simulink model "fmpc_simulation_3modelle"  (R2022b)
settings: Solver=VariableStepAuto  StartTime=0.0  StopTime=T  RelTol=1e-7
undefined symbols (not defined in the file): Am, b, Bm, c_1, c_2, C_hilf, Cm, D, dt, F1, F2, F3, fuzzy_menge, H1, H2, H3, PhiU1, PhiU2, PhiU3, PhiZ1, PhiZ2, PhiZ3, Qy1, Qy2, Qy3
settings Model: Creator=benja  LastModifiedBy=benja

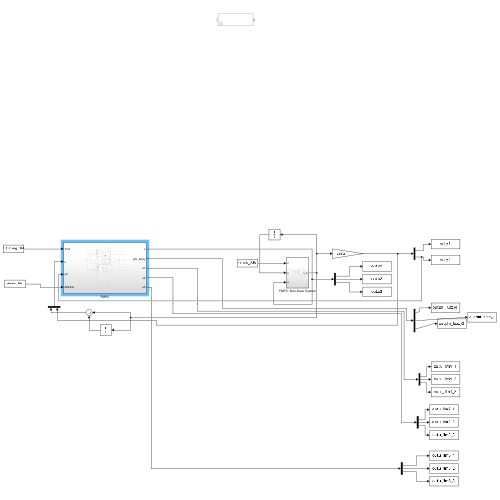
[thumbnail: Simulink's stored preview of the top-level diagram]
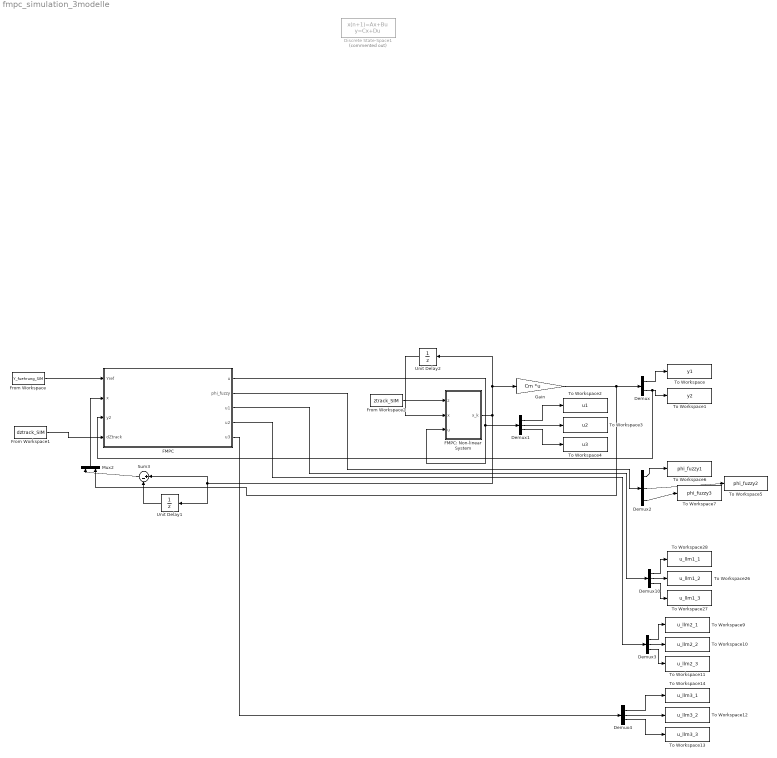
== system fmpc_simulation_3modelle ==
  Demux : Demux  Outputs=2
  Demux{1..4,10} (5 alike) : Demux  Outputs=3
  Discrete State-Space1 : DiscreteStateSpace  Commented=on  A=Am  B=Bm  C=C_hilf  D=D  SampleTime=dt
  FMPC : Subsystem
  FMPC: Non-linear System : Subsystem
  From Workspace : FromWorkspace  VariableName=Y_fuehrung_SIM  OutDataTypeStr=double  SampleTime=dt
  From Workspace1 : FromWorkspace  VariableName=dztrack_SIM  OutDataTypeStr=double  SampleTime=dt
  From Workspace2 : FromWorkspace  VariableName=ztrack_SIM  OutDataTypeStr=double  SampleTime=dt
  Gain : Gain  Gain=Cm  Multiplication=Matrix(K*u)
  Mux2 : Mux  Inputs=2
  Sum3 : Sum  Inputs=|+-
  To Workspace : ToWorkspace  VariableName=y1  SampleTime=-1
      settings: Save2DSignal=2-D array (concatenate along first dimension)
  To Workspace1 : ToWorkspace  VariableName=y2  SampleTime=-1
      settings: Save2DSignal=2-D array (concatenate along first dimension)
  To Workspace10 : ToWorkspace  VariableName=u_llm2_2  SampleTime=-1
      settings: Save2DSignal=2-D array (concatenate along first dimension)
  To Workspace11 : ToWorkspace  VariableName=u_llm2_3  SampleTime=-1
      settings: Save2DSignal=2-D array (concatenate along first dimension)
  To Workspace12 : ToWorkspace  VariableName=u_llm3_2  SampleTime=-1
      settings: Save2DSignal=2-D array (concatenate along first dimension)
  To Workspace13 : ToWorkspace  VariableName=u_llm3_3  SampleTime=-1
      settings: Save2DSignal=2-D array (concatenate along first dimension)
  To Workspace14 : ToWorkspace  VariableName=u_llm3_1  SampleTime=-1
      settings: Save2DSignal=2-D array (concatenate along first dimension)
  To Workspace2 : ToWorkspace  VariableName=u1  SampleTime=-1
      settings: Save2DSignal=2-D array (concatenate along first dimension)
  To Workspace26 : ToWorkspace  VariableName=u_llm1_2  SampleTime=-1
      settings: Save2DSignal=2-D array (concatenate along first dimension)
  To Workspace27 : ToWorkspace  VariableName=u_llm1_3  SampleTime=-1
      settings: Save2DSignal=2-D array (concatenate along first dimension)
  To Workspace28 : ToWorkspace  VariableName=u_llm1_1  SampleTime=-1
      settings: Save2DSignal=2-D array (concatenate along first dimension)
  To Workspace3 : ToWorkspace  VariableName=u2  SampleTime=-1
      settings: Save2DSignal=2-D array (concatenate along first dimension)
  To Workspace4 : ToWorkspace  VariableName=u3  SampleTime=-1
      settings: Save2DSignal=2-D array (concatenate along first dimension)
  To Workspace5 : ToWorkspace  VariableName=phi_fuzzy2  SampleTime=-1
      settings: Save2DSignal=2-D array (concatenate along first dimension)
  To Workspace6 : ToWorkspace  VariableName=phi_fuzzy1  SampleTime=-1
      settings: Save2DSignal=2-D array (concatenate along first dimension)
  To Workspace7 : ToWorkspace  VariableName=phi_fuzzy3  SampleTime=-1
      settings: Save2DSignal=2-D array (concatenate along first dimension)
  To Workspace9 : ToWorkspace  VariableName=u_llm2_1  SampleTime=-1
      settings: Save2DSignal=2-D array (concatenate along first dimension)
  Unit Delay1 : UnitDelay  SampleTime=-1  HasFrameUpgradeWarning=on
  Unit Delay2 : UnitDelay  SampleTime=-1  HasFrameUpgradeWarning=on
  wires:
  Demux/1 -> To Workspace/1
  Demux1/1 -> To Workspace2/1
  Demux1/2 -> To Workspace3/1
  Unit Delay1/1 -> Sum3/2
  Gain/1 -> Demux/1, Mux2/2
  Sum3/1 -> Mux2/1
  Demux1/3 -> To Workspace4/1
  FMPC: Non-linear System/1(x_k) -> Unit Delay2/1, Gain/1, Sum3/1, Unit Delay1/1
  Unit Delay2/1 -> FMPC: Non-linear System/2(x)
  FMPC/1(u) -> FMPC: Non-linear System/3(u), Demux1/1
  From Workspace/1 -> FMPC/1(Yref)
  Mux2/1 -> FMPC/2(x)
  FMPC/2(phi_fuzzy) -> Demux2/1
  Demux2/1 -> To Workspace6/1
  Demux2/2 -> To Workspace5/1
  Demux2/3 -> To Workspace7/1
  Demux/2 -> FMPC/3(y2), To Workspace1/1
  Demux3/3 -> To Workspace11/1
  Demux3/2 -> To Workspace10/1
  FMPC/4(u2) -> Demux3/1
  Demux3/1 -> To Workspace9/1
  Demux4/1 -> To Workspace14/1
  FMPC/5(u3) -> Demux4/1
  Demux4/2 -> To Workspace12/1
  Demux4/3 -> To Workspace13/1
  Demux10/2 -> To Workspace26/1
  Demux10/3 -> To Workspace27/1
  Demux10/1 -> To Workspace28/1
  FMPC/3(u1) -> Demux10/1
  From Workspace2/1 -> FMPC: Non-linear System/1(z)
  From Workspace1/1 -> FMPC/4(dZtrack)

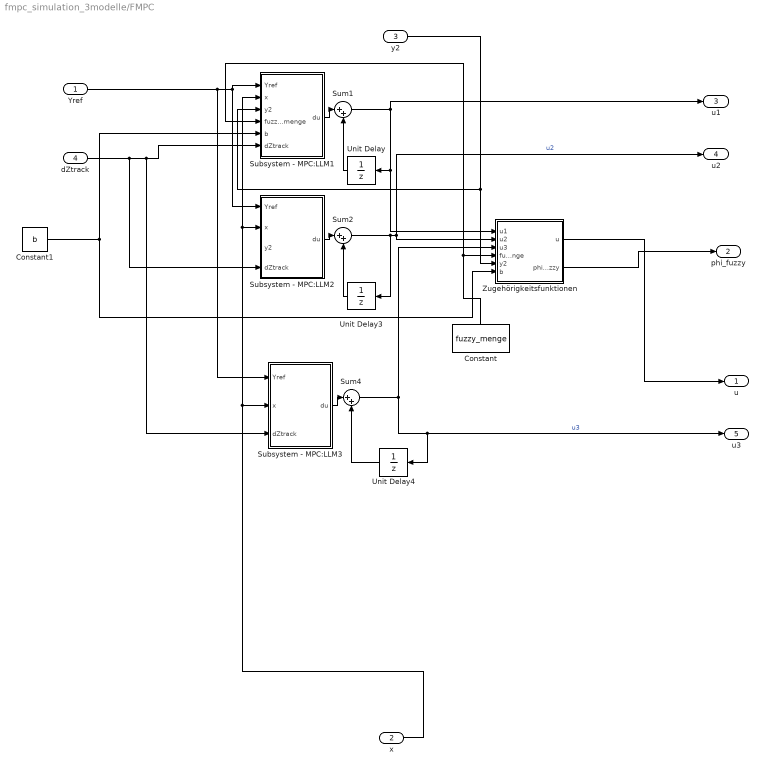
== system fmpc_simulation_3modelle/FMPC ==
  Yref : Inport
  x : Inport  Port=2
  y2 : Inport  Port=3
  dZtrack : Inport  Port=4
  Constant : Constant  Value=fuzzy_menge
  Constant1 : Constant  Value=b
  Subsystem - MPC:LLM1 : Subsystem
  Subsystem - MPC:LLM2 : Subsystem
  Subsystem - MPC:LLM3 : Subsystem
  Sum1 : Sum  Inputs=|++
  Sum2 : Sum  Inputs=|++
  Sum4 : Sum  Inputs=|++
  Unit Delay : UnitDelay  SampleTime=dt  HasFrameUpgradeWarning=on
  Unit Delay3 : UnitDelay  SampleTime=dt  HasFrameUpgradeWarning=on
  Unit Delay4 : UnitDelay  SampleTime=dt  HasFrameUpgradeWarning=on
  Zugehörigkeitsfunktionen : MATLAB Function  TreatAsAtomicUnit=on
  u : Outport
  phi_fuzzy : Outport  Port=2
  u1 : Outport  Port=3
  u2 : Outport  Port=4
  u3 : Outport  Port=5
  wires:
  Sum4/1 -> u3/1, Unit Delay4/1, Zugehörigkeitsfunktionen/3(u3)  "u3"
  Sum2/1 -> Unit Delay3/1, u2/1, Zugehörigkeitsfunktionen/2(u2)  "u2"
  Zugehörigkeitsfunktionen/1(u) -> u/1
  Subsystem - MPC:LLM3/1(du) -> Sum4/1
  x/1 -> Subsystem - MPC:LLM1/2(x), Subsystem - MPC:LLM2/2(x), Subsystem - MPC:LLM3/2(x)
  Yref/1 -> Subsystem - MPC:LLM1/1(Yref), Subsystem - MPC:LLM2/1(Yref), Subsystem - MPC:LLM3/1(Yref)
  Subsystem - MPC:LLM1/1(du) -> Sum1/1
  Subsystem - MPC:LLM2/1(du) -> Sum2/1
  Sum1/1 -> Zugehörigkeitsfunktionen/1(u1), Unit Delay/1, u1/1
  Unit Delay/1 -> Sum1/2
  Unit Delay3/1 -> Sum2/2
  Constant/1 -> Zugehörigkeitsfunktionen/4(fuzzy_menge), Subsystem - MPC:LLM1/4(fuzzy_menge)
  Zugehörigkeitsfunktionen/2(phi_fuzzy) -> phi_fuzzy/1
  Constant1/1 -> Subsystem - MPC:LLM1/5(b), Zugehörigkeitsfunktionen/6(b)
  y2/1 -> Zugehörigkeitsfunktionen/5(y2), Subsystem - MPC:LLM1/3(y2)
  Unit Delay4/1 -> Sum4/2
  dZtrack/1 -> Subsystem - MPC:LLM2/4(dZtrack), Subsystem - MPC:LLM3/3(dZtrack), Subsystem - MPC:LLM1/6(dZtrack)

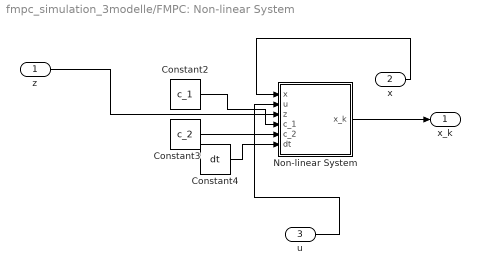
== system fmpc_simulation_3modelle/FMPC: Non-linear System ==
  z : Inport
  x : Inport  Port=2
  u : Inport  Port=3
  Constant2 : Constant  Value=c_1
  Constant3 : Constant  Value=c_2
  Constant4 : Constant  Value=dt
  Non-linear System : MATLAB Function  TreatAsAtomicUnit=on
  x_k : Outport
  wires:
  x/1 -> Non-linear System/1(x)
  Constant3/1 -> Non-linear System/5(c_2)
  Constant4/1 -> Non-linear System/6(dt)
  u/1 -> Non-linear System/2(u)
  Constant2/1 -> Non-linear System/4(c_1)
  z/1 -> Non-linear System/3(z)
  Non-linear System/1(x_k) -> x_k/1

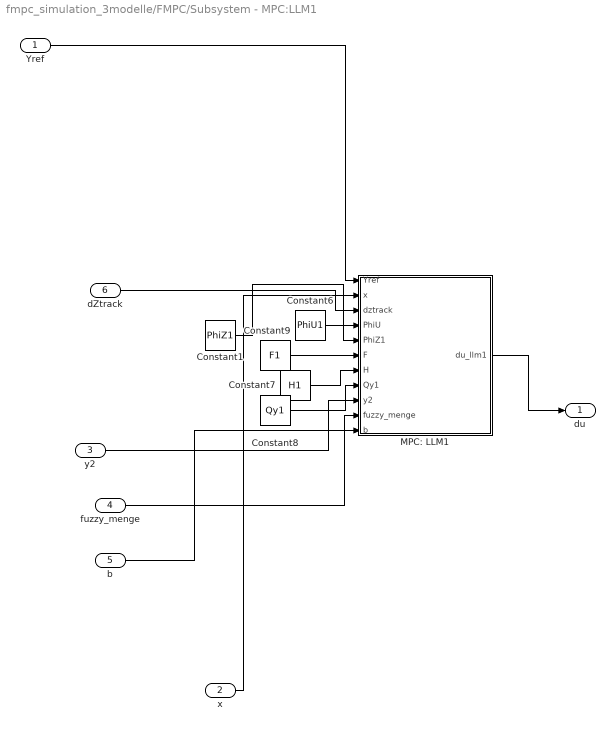
== system fmpc_simulation_3modelle/FMPC/Subsystem - MPC:LLM1 ==
  Yref : Inport
  x : Inport  Port=2
  y2 : Inport  Port=3
  fuzzy_menge : Inport  Port=4
  b : Inport  Port=5
  dZtrack : Inport  Port=6
  Constant1 : Constant  Value=PhiZ1  SampleTime=dt
  Constant6 : Constant  Value=PhiU1  SampleTime=dt
  Constant7 : Constant  Value=H1  SampleTime=dt
  Constant8 : Constant  Value=Qy1  SampleTime=dt
  Constant9 : Constant  Value=F1  SampleTime=dt
  MPC: LLM1 : MATLAB Function  TreatAsAtomicUnit=on
  du : Outport
  wires:
  Constant7/1 -> MPC: LLM1/7(H)
  Constant9/1 -> MPC: LLM1/6(F)
  x/1 -> MPC: LLM1/2(x)
  Yref/1 -> MPC: LLM1/1(Yref)
  MPC: LLM1/1(du_llm1) -> du/1
  Constant8/1 -> MPC: LLM1/8(Qy1)
  Constant6/1 -> MPC: LLM1/4(PhiU)
  y2/1 -> MPC: LLM1/9(y2)
  fuzzy_menge/1 -> MPC: LLM1/10(fuzzy_menge)
  b/1 -> MPC: LLM1/11(b)
  dZtrack/1 -> MPC: LLM1/3(dztrack)
  Constant1/1 -> MPC: LLM1/5(PhiZ1)

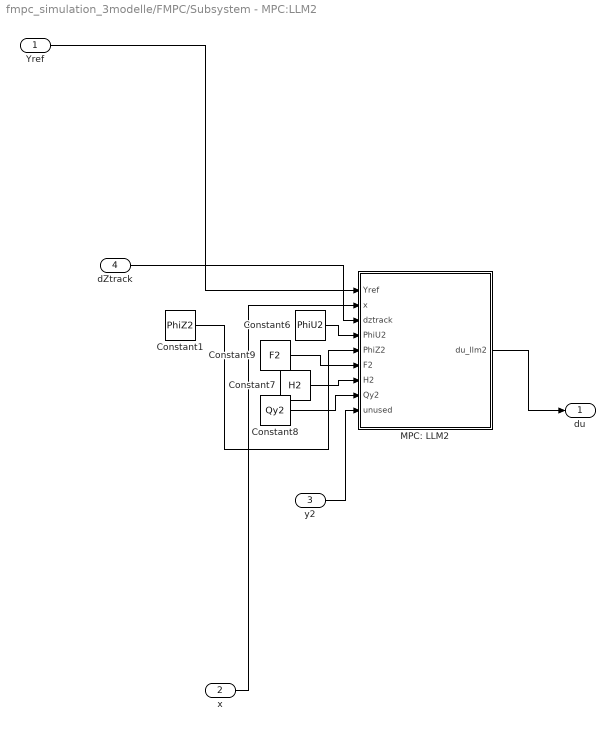
== system fmpc_simulation_3modelle/FMPC/Subsystem - MPC:LLM2 ==
  Yref : Inport
  x : Inport  Port=2
  y2 : Inport  Port=3
  dZtrack : Inport  Port=4
  Constant1 : Constant  Value=PhiZ2  SampleTime=dt
  Constant6 : Constant  Value=PhiU2  SampleTime=dt
  Constant7 : Constant  Value=H2  SampleTime=dt
  Constant8 : Constant  Value=Qy2  SampleTime=dt
  Constant9 : Constant  Value=F2  SampleTime=dt
  MPC: LLM2 : MATLAB Function  TreatAsAtomicUnit=on
  du : Outport
  wires:
  Constant7/1 -> MPC: LLM2/7(H2)
  Constant9/1 -> MPC: LLM2/6(F2)
  x/1 -> MPC: LLM2/2(x)
  Constant6/1 -> MPC: LLM2/4(PhiU2)
  Yref/1 -> MPC: LLM2/1(Yref)
  MPC: LLM2/1(du_llm2) -> du/1
  Constant8/1 -> MPC: LLM2/8(Qy2)
  Constant1/1 -> MPC: LLM2/5(PhiZ2)
  y2/1 -> MPC: LLM2/9(unused)
  dZtrack/1 -> MPC: LLM2/3(dztrack)

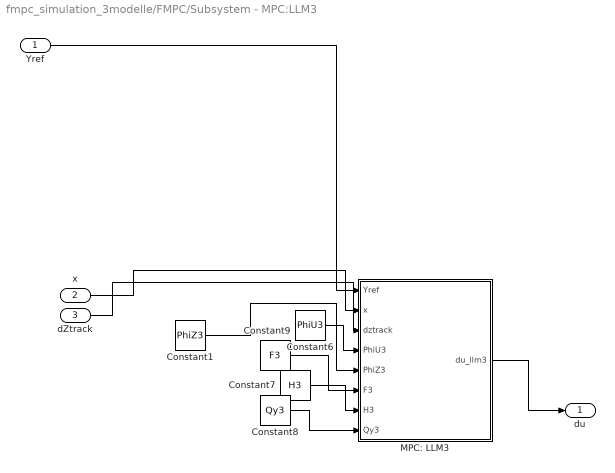
== system fmpc_simulation_3modelle/FMPC/Subsystem - MPC:LLM3 ==
  Yref : Inport
  x : Inport  Port=2
  dZtrack : Inport  Port=3
  Constant1 : Constant  Value=PhiZ3  SampleTime=dt
  Constant6 : Constant  Value=PhiU3  SampleTime=dt
  Constant7 : Constant  Value=H3  SampleTime=dt
  Constant8 : Constant  Value=Qy3  SampleTime=dt
  Constant9 : Constant  Value=F3  SampleTime=dt
  MPC: LLM3 : MATLAB Function  TreatAsAtomicUnit=on
  du : Outport
  wires:
  Constant7/1 -> MPC: LLM3/7(H3)
  Constant9/1 -> MPC: LLM3/6(F3)
  x/1 -> MPC: LLM3/2(x)
  Constant6/1 -> MPC: LLM3/4(PhiU3)
  Yref/1 -> MPC: LLM3/1(Yref)
  MPC: LLM3/1(du_llm3) -> du/1
  Constant8/1 -> MPC: LLM3/8(Qy3)
  Constant1/1 -> MPC: LLM3/5(PhiZ3)
  dZtrack/1 -> MPC: LLM3/3(dztrack)

== matlab function fmpc_simulation_3modelle/FMPC: Non-linear System/Non-linear System ==
  data: x input size=[4 1]; u input size=[3 1]; z input size=1; x_k output size=[4 1]; c_1 input size=1; c_2 input size=1; dt input size=1
function x_k = fcn(x,u,z,c_1,c_2,dt)
    
    g_RS = 2.6;   
    r_3  = 0.3;   
    r_2 = r_3 / g_RS;    
    r_1 = (r_2 + r_3)/2; 
    r_p = r_3-r_2;
    r_Wheel=0.3;
    g_TT = 66/54*80/23;

    d_s  = 0.096;
    m_p  = 1*4;    
    m_car = 1300;

    J_1  = .1;      
    J_2  = 0.03;     
    J_3  = 0.1;     
    J_p  = 0.01*4;   
    J_4  = m_car*r_Wheel^2 / g_TT^2;  

    M_1 = J_1 + J_2 * 4 * r_1^2/r_2^2 + J_p * r_1^2/r_p^2 + m_p * r_1^2;
    M_2 = J_2 * 2 * r_1 * r_3 / r_2^2 + J_p * r_1 * r_3 / r_p^2;
    M_4 = J_2 * r_3^2 / r_2^2 + J_3 + J_p * r_3^2 / r_p^2;
    M_3 = J_2 * ( (2 * r_1 * r_3 ) / r_2 ^ 2 ) + J_p*((r_1 * r_3) / r_p^2);
    M_5 = M_4 - M_2*M_3/M_1;
    
%     x_k1 = x(3) - x(4);
%     
%     x_k2 = -(M_2/(M_5*M_1)) * ...
%         (c_1*x(4)^2+c_2)*x(1) ... 
%         - (M_2/(M_5*M_1))*d_s*x(3) ...
%         + (M_2/(M_5*M_1))*d_s*x(4) ...
%         + (1+((M_2*M_3)/(M_1*M_5)))/M_1*u(1) ...
%         + ((2*r_1/r_2) + (M_2/M_5)*(2*r_1*M_3/(r_2*M_1) - (r_3/r_2)))/M_1 * u(2) ...
%         + M_2/(M_5*M_1)*u(3);
%     
%     x_k3 = -(1/M_5)*(c_1*x(4)^2+c_2)*x(1)...
%         - (1/M_5)*d_s*x(3) + (1/M_5)*d_s*x(4) + ...
%         M_3/(M_1*M_5)*u(1) + ((2*r_1 * M_3)/(r_2*M_1)-r_3/r_2)/M_5*u(2) + (1/M_5) * u(3); 
%     
%     x_k4 = (1/J_4)*(c_1*x(4)^2+c_2)*x(1) ... 
%         + (1/J_4)*(d_s)*x(3) - (1/J_4)*(d_s) * x(4) - (1/J_4) * z;
% 
%     x_k = x + [x_k1;x_k2;x_k3;x_k4]*dt;



 
    k11 = x(3) - x(4);

    k12 = -(M_2 / (M_5 * M_1)) * (c_1 * x(4)^2 + c_2)*x(1) ...
        - (M_2 / (M_5 * M_1)) * d_s * x(3) ...
        + (M_2 / (M_5 * M_1)) * d_s * x(4) ...
        + (1 + ((M_2 * M_3) / (M_1 * M_5))) * u(1) ...
        + ((2 * r_1 / r_2) + (M_2 / M_5) * (2 *r_1 * M_3 / (r_2 * M_1) - (r_3 / r_2))) / M_1 * u(2) ...
        + M_2 / (M_5 * M_1) * u(3);
    
    k13 = -(1 / M_5) * (c_1 * x(4)^2 + c_2) * x(1) - (1 / M_5) * d_s * x(3) + (1 / M_5) * d_s * x(4) + ...
        M_3 / (M_1 * M_5) * u(1) + ((2 * r_1 * M_3) / (r_2 * M_1) - r_3 / r_2) / M_5 * u(2) + (1 / M_5) * u(3);

    k14 = (1 / J_4) * (c_1 * x(4)^2 + c_2) * x(1) + (1 / J_4)*(d_s) * x(3) - ( 1 / J_4) * (d_s) * x(4) - (1 / J_4) * z;
 

    k21 = (x(3) + k13 * dt / 2) - (x(4) + k14 * dt / 2);

    k22 = -(M_2 / (M_5 * M_1)) * (c_1 * (x(4) + k14 * dt / 2)^2 + c_2) * (x(1) + k11 * dt / 2) ...
        - (M_2 / (M_5 * M_1)) * d_s * (x(3) + k13 * dt / 2) ...
        + (M_2 / (M_5 * M_1)) * d_s * (x(4) + k14 * dt / 2) ...
        + (1+ ((M_2 * M_3) / (M_1 * M_5))) * u(1) ...
        + ((2 * r_1 / r_2) + (M_2 / M_5) * ( 2 * r_1 * M_3 / (r_2 * M_1) - (r_3 / r_2))) / M_1 * u(2) ...
        + M_2 / (M_5 * M_1) * u(3);
        
    k23 = -(1 / M_5) * (c_1 * (x(4) + k14 * dt / 2)^2+c_2)*(x(1) + k11 * dt / 2) ...
        - (1 / M_5) * d_s * (x(3) + k13 * dt / 2) ...
        + (1 / M_5) * d_s * ( x(4) + k14 * dt / 2) ...
        + M_3 / (M_1 * M_5) * u(1) ...
        + ((2 * r_1 * M_3) / (r_2 * M_1) - r_3 / r_2) / M_5 * u(2) ...
        + (1 / M_5) * u(3);
    
    k24 = (1 / J_4) * (c_1 * (x(4) + k14 * dt / 2)^2 + c_2)*(x(1) + k11 * dt / 2) ...
        + (1 / J_4) * (d_s) * (x(3) + k13 * dt / 2) ...
        - (1 / J_4) * (d_s) * (x(4) + k14 * dt / 2) ...
        - (1 / J_4) * z;
   

    k31 = (x(3) + k23 * dt / 2) - (x(4) + k24 * dt / 2);

    k32 = -(M_2 / (M_5 * M_1)) * (c_1 * (x(4) + k24 * dt / 2)^2 + c_2) * (x(1) + k21 * dt / 2) ...
        - (M_2 / (M_5 * M_1)) * d_s * (x(3) + k23 * dt / 2) ...
        + (M_2 / (M_5 * M_1)) * d_s * (x(4) + k24 * dt / 2) ...
        + (1 + ((M_2 * M_3) / (M_1 * M_5))) * u(1) ...
        + ((2 * r_1 / r_2) + (M_2 / M_5) * (2 * r_1 * M_3 / (r_2 * M_1) - (r_3 / r_2))) / M_1 * u(2) ...
        + M_2 / (M_5 * M_1) * u(3);
    
    k33 = -(1 / M_5)*(c_1 * (x(4) + k24 * dt / 2)^2 + c_2) * (x(1) + k21 * dt / 2) ...
        - (1 / M_5) * d_s * (x(3) + k23 * dt / 2) ...
        + (1 / M_5) * d_s * (x(4) + k24 * dt / 2) ...
        + M_3 / (M_1 * M_5) * u(1) ...
        + ((2 * r_1 * M_3) / (r_2 * M_1) - r_3 / r_2) / M_5 * u(2) ...
        + (1 / M_5) * u(3);
    
    k34 = (1 / J_4) * (c_1 * (x(4) + k24 * dt / 2)^2 + c_2) * (x(1) + k21 * dt / 2) ...
        + (1 / J_4) * (d_s) * (x(3) + k23 * dt /2) ...
        - (1 / J_4) * (d_s) * (x(4) + k24 * dt / 2) ...
        - (1 / J_4) * z;
    

    k41 = (x(3) + k33 * dt) - (x(4) + k34 * dt);

    k42 = -(M_2 / (M_5 * M_1)) * (c_1 * (x(4) + k34 * dt)^2 + c_2) * (x(1) + k31 * dt) ...
        - (M_2 / (M_5 * M_1)) * d_s * (x(3) + k33 * dt ) ...
        + (M_2 / (M_5 * M_1)) * d_s * (x(4) + k34 * dt ) ...
        + (1 + ((M_2 * M_3) / (M_1 * M_5))) * u(1) ...
        + ((2 * r_1 / r_2) + (M_2 / M_5) * (2 * r_1 * M_3 / (r_2 * M_1) - (r_3 / r_2))) / M_1 * u(2) ...
        + M_2 / (M_5 * M_1) * u(3);
    
    k43 = -(1 / M_5) * (c_1 * (x(4) + k34 * dt)^2 + c_2) * (x(1) + k31 * dt ) ...
        - (1 / M_5) * d_s * (x(3) + k33 * dt ) ...
        + (1 / M_5) * d_s * (x(4) + k34 * dt ) ...
        + M_3 / (M_1 * M_5) * u(1) ...
        + ((2 * r_1 * M_3)/(r_2 * M_1) - r_3 / r_2) / M_5 * u(2) ...
        + (1 / M_5) * u(3);
    
    k44 = (1 / J_4) * (c_1 * (x(4) + k34 * dt )^2 + c_2) * (x(1) + k31 * dt ) ...
        + (1 / J_4) * (d_s) * (x(3) + k33 * dt ) ...
        - (1 / J_4) * (d_s) * (x(4) + k34 * dt ) ...
        - (1 / J_4) * z;

    x_k = x + dt * ([k11;k12;k13;k14] + 2 * [k21;k22;k23;k24] + 2 * [k31;k32;k33;k34] + [k41;k42;k43;k44]) / 6;

== matlab function fmpc_simulation_3modelle/FMPC/Subsystem - MPC:LLM1/MPC: LLM1 ==
  data: Yref input size=[100 1]; du_llm1 output size=[3 1]; x input size=[6 1]; dztrack input; PhiU input size=[100 45]; PhiZ1 input; F input size=[100 6]; H input size=[45 45]; Qy1 input size=[100 100]; y2 input; fuzzy_menge input size=[2 2]; b input
function du_llm1 = fcn(Yref,x,dztrack,PhiU,PhiZ1,F,H,Qy1,y2,fuzzy_menge,b)
    nu = 3;
    if y2 <= fuzzy_menge(1,2)-b
        f = -PhiU' * Qy1 * ( Yref - F*x - PhiZ1*dztrack);
        dU = -H\f; % -inv(H)*f
        du_llm1 = dU(1:nu,1);
    else
        du_llm1 = zeros(nu,1);
    end
    
end

== matlab function fmpc_simulation_3modelle/FMPC/Subsystem - MPC:LLM2/MPC: LLM2 ==
  data: Yref input size=[100 1]; du_llm2 output size=[3 1]; x input size=[6 1]; dztrack input; PhiU2 input size=[100 45]; PhiZ2 input; F2 input size=[100 6]; H2 input size=[45 45]; Qy2 input size=[100 100]; unused input
function du_llm2 = fcn(Yref,x,dztrack,PhiU2,PhiZ2,F2,H2,Qy2,~)
    nu = 3;
    f = -PhiU2' * Qy2 * ( Yref - F2*x - PhiZ2*dztrack);
    dU = -H2\f; % -inv(H)*f
    du_llm2 = dU(1:nu,1);
    
end

== matlab function fmpc_simulation_3modelle/FMPC/Subsystem - MPC:LLM3/MPC: LLM3 ==
  data: Yref input size=[100 1]; du_llm3 output size=[3 1]; x input size=[6 1]; dztrack input size=[50 1]; PhiU3 input size=[100 45]; PhiZ3 input size=[100 50]; F3 input size=[100 6]; H3 input size=[45 45]; Qy3 input size=[100 100]
function du_llm3 = fcn(Yref,x,dztrack,PhiU3,PhiZ3,F3,H3,Qy3)
    nu = 3;
    f3 = -PhiU3' * Qy3 * ( Yref - F3*x - PhiZ3*dztrack);
    dU = -H3\f3; % -inv(H)*f
    du_llm3 = dU(1:nu,1);
    
end

== matlab function fmpc_simulation_3modelle/FMPC/Zugehörigkeitsfunktionen ==
  data: u1 input size=[3 1]; u output size=[3 1]; u2 input size=[3 1]; u3 input size=[3 1]; fuzzy_menge input size=[2 2]; y2 input size=1; phi_fuzzy output size=[3 1]; b input size=1
function [u,phi_fuzzy] = fcn(u1,u2,u3,fuzzy_menge,y2,b)
    %% 3x Modelle
  phi_fuzzy1 = trapmf(y2,[-100000000,-100000000,fuzzy_menge(1,1)+b,fuzzy_menge(1,2)-b]);
  phi_fuzzy2 = trapmf(y2,[fuzzy_menge(1,1)+b,fuzzy_menge(1,2)-b,fuzzy_menge(1,2)+b,fuzzy_menge(2,2)-b]);
  phi_fuzzy3 = trapmf(y2,[fuzzy_menge(1,2)+b,fuzzy_menge(2,2)-b,100000000,100000000]);

    u = (u1 * phi_fuzzy1 + u2 * phi_fuzzy2 + u3 * phi_fuzzy3)/(phi_fuzzy1+phi_fuzzy2+phi_fuzzy3);
    phi_fuzzy = [phi_fuzzy1; phi_fuzzy2; phi_fuzzy3];

    %% 4x Modelle
%         phi_fuzzy1 = trapmf(y2,[-100000000,-100000000,fuzzy_menge(1,1)+b,fuzzy_menge(1,2)-b]);
%         phi_fuzzy2 = trapmf(y2,[fuzzy_menge(1,1)+b,fuzzy_menge(1,2)-b,fuzzy_menge(1,2)+b,fuzzy_menge(2,2)-b]);
%         phi_fuzzy3 = trapmf(y2,[fuzzy_menge(1,2)+b,fuzzy_menge(2,2)-b,fuzzy_menge(2,2)+b,fuzzy_menge(3,2)-b]);
%         phi_fuzzy4 = trapmf(y2,[fuzzy_menge(2,2)+b,fuzzy_menge(3,2)-b,100000000,100000000]);
% 
%     u = (u1 * phi_fuzzy1 + u2 * phi_fuzzy2 + u3 * phi_fuzzy3 + u4 * phi_fuzzy4)/(phi_fuzzy1+phi_fuzzy2+phi_fuzzy3+phi_fuzzy4);
%     phi_fuzzy = [phi_fuzzy1; phi_fuzzy2; phi_fuzzy3; phi_fuzzy4];
